simulink model "Hunter_Real_call"  (R2023a)
settings: Solver=ode3  StartTime=0.0  StopTime=inf  FixedStep=0.05  RelTol=1e-3  EnableMultiTasking=on
InitFcn:
  | rosshutdown
  | rosinit("http://localhost:11311")
model workspace (MAT data in the model file):
  SL_ROS_VariableLengthArrays_MaxSizes.CommonInfo.ArrayTruncateAction = 'EmitWarning'
  SL_ROS_VariableLengthArrays_MaxSizes.MsgTypeMap = containers.Map
  SL_ROS_VariableLengthArrays_MaxSizes.MsgTypeMap.serialization.keys = {'cob_object_detection_msgs/Detection', 'cob_object_detection_msgs/DetectionArray', 'gazebo_msgs/ModelStates', 'sensor_msgs/PointCloud2'}
  SL_ROS_VariableLengthArrays_MaxSizes.MsgTypeMap.serialization.values{1}(1).PropertyName = 'Detector'
  SL_ROS_VariableLengthArrays_MaxSizes.MsgTypeMap.serialization.values{1}(1).DataType = 'uint8'
  SL_ROS_VariableLengthArrays_MaxSizes.MsgTypeMap.serialization.values{1}(1).MaxLength = 128
  SL_ROS_VariableLengthArrays_MaxSizes.MsgTypeMap.serialization.values{1}(2).PropertyName = 'Label'
  SL_ROS_VariableLengthArrays_MaxSizes.MsgTypeMap.serialization.values{1}(2).DataType = 'uint8'
  SL_ROS_VariableLengthArrays_MaxSizes.MsgTypeMap.serialization.values{1}(2).MaxLength = 128
  SL_ROS_VariableLengthArrays_MaxSizes.MsgTypeMap.serialization.values{2}.PropertyName = 'Detections'
  SL_ROS_VariableLengthArrays_MaxSizes.MsgTypeMap.serialization.values{2}.DataType = 'cob_object_detection_msgs/Detection'
  SL_ROS_VariableLengthArrays_MaxSizes.MsgTypeMap.serialization.values{2}.MaxLength = 100
  SL_ROS_VariableLengthArrays_MaxSizes.MsgTypeMap.serialization.values{3}(1).PropertyName = 'Name'
  SL_ROS_VariableLengthArrays_MaxSizes.MsgTypeMap.serialization.values{3}(1).DataType = 'std_msgs/String'
  SL_ROS_VariableLengthArrays_MaxSizes.MsgTypeMap.serialization.values{3}(1).MaxLength = 266
  SL_ROS_VariableLengthArrays_MaxSizes.MsgTypeMap.serialization.values{3}(2).PropertyName = 'Pose'
  SL_ROS_VariableLengthArrays_MaxSizes.MsgTypeMap.serialization.values{3}(2).DataType = 'geometry_msgs/Pose'
  SL_ROS_VariableLengthArrays_MaxSizes.MsgTypeMap.serialization.values{3}(2).MaxLength = 350
  SL_ROS_VariableLengthArrays_MaxSizes.MsgTypeMap.serialization.values{3}(3).PropertyName = 'Twist'
  SL_ROS_VariableLengthArrays_MaxSizes.MsgTypeMap.serialization.values{3}(3).DataType = 'geometry_msgs/Twist'
  SL_ROS_VariableLengthArrays_MaxSizes.MsgTypeMap.serialization.values{3}(3).MaxLength = 350
  SL_ROS_VariableLengthArrays_MaxSizes.MsgTypeMap.serialization.values{4}(1).PropertyName = 'Data'
  SL_ROS_VariableLengthArrays_MaxSizes.MsgTypeMap.serialization.values{4}(1).DataType = 'uint8'
  SL_ROS_VariableLengthArrays_MaxSizes.MsgTypeMap.serialization.values{4}(1).MaxLength = 1050000
  SL_ROS_VariableLengthArrays_MaxSizes.MsgTypeMap.serialization.values{4}(2).PropertyName = 'Fields'
  SL_ROS_VariableLengthArrays_MaxSizes.MsgTypeMap.serialization.values{4}(2).DataType = 'sensor_msgs/PointField'
  SL_ROS_VariableLengthArrays_MaxSizes.MsgTypeMap.serialization.values{4}(2).MaxLength = 1000
  SL_ROS_VariableLengthArrays_MaxSizes.MsgTypeMap.serialization.uniformity = 0
  SL_ROS_VariableLengthArrays_MaxSizes.MsgTypeMap.serialization.keyType = 'char'
  SL_ROS_VariableLengthArrays_MaxSizes.MsgTypeMap.serialization.valueType = 'any'
undefined symbols (not defined in the file or in its folder): Angular, L, Ld, Linear
libraries: robotlib x10, slpidlib x2, slctrlblks x1, robotalgslib x1, mobileRoboticsLib x1, robotcorelib x1
settings Model: Creator=aiv_  LastModifiedBy=aiv
settings SolverCC: AutoInsertRateTranBlk=on
settings DataIOCC: SaveFormat=Array  ReturnWorkspaceOutputs=off
settings OptimizationCC: EnhancedBackFolding=on  PassReuseOutputArgsAs=Individual arguments  StateBitsets=on  DataBitsets=on  ZeroExternalMemoryAtStartup=off  ZeroInternalMemoryAtStartup=off  NoFixptDivByZeroProtection=on  LifeSpan=1  MaxStackSize=64  OptimizeBlockOrder=speed  DifferentSizesBufferReuse=on  EfficientTunableParamExpr=on
settings DebuggingCC: ParameterTunabilityLossMsg=error
settings HardwareCC: ProdBitPerPointer=32  ProdBitPerSizeT=32  ProdBitPerPtrDiffT=32  ProdLargestAtomicFloat=None  ProdWordSize=32  ProdHWDeviceType=Custom Processor->Custom Processor
settings ModelReferenceCC: PropagateSignalLabelsOutOfModel=off
settings SFSimCC: SimTargetLang=C++
settings RTWCC: Description=Embedded Coder  SystemTargetFile=ert.tlc  HardwareBoard=Robot Operating System (ROS)  TLCOptions=-p0 -aRateBasedStepFcn=0  TemplateMakefile=ert_default_tmf  GenerateReport=on  RTWVerbose=off  Toolchain=Catkin  IncludeHyperlinkInReport=on  LaunchReport=on  TargetLang=C++
settings CodeAppCC: ForceParamTrailComments=on  IgnoreCustomStorageClasses=off  OperatorAnnotations=on  SimulinkDataObjDesc=on  SFDataObjDesc=on  CustomSymbolStrGlobalVar=rt$N$M  CustomSymbolStrType=$N$M  CustomSymbolStrFcn=$N$M$F  CustomSymbolStrMacro=$N$M  InsertBlockDesc=on
settings ERTTargetCC: CodeReplacementLibrary=GNU C99 extensions  SuppressErrorStatus=on  CodeInterfacePackaging=C++ class  SupportVariableSizeSignals=on  RootIOFormat=Structure reference  ERTCustomFileTemplate=example_file_process.tlc

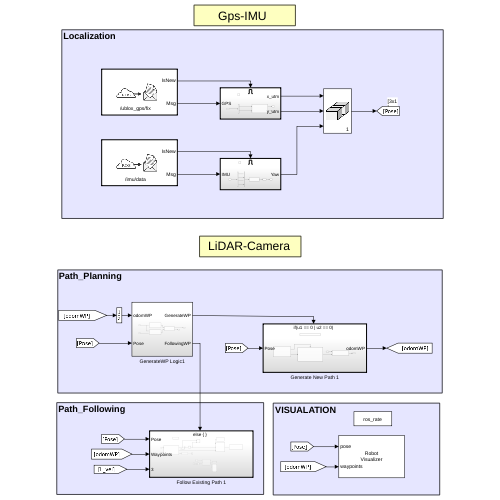
[thumbnail: Simulink's stored preview of the top-level diagram]
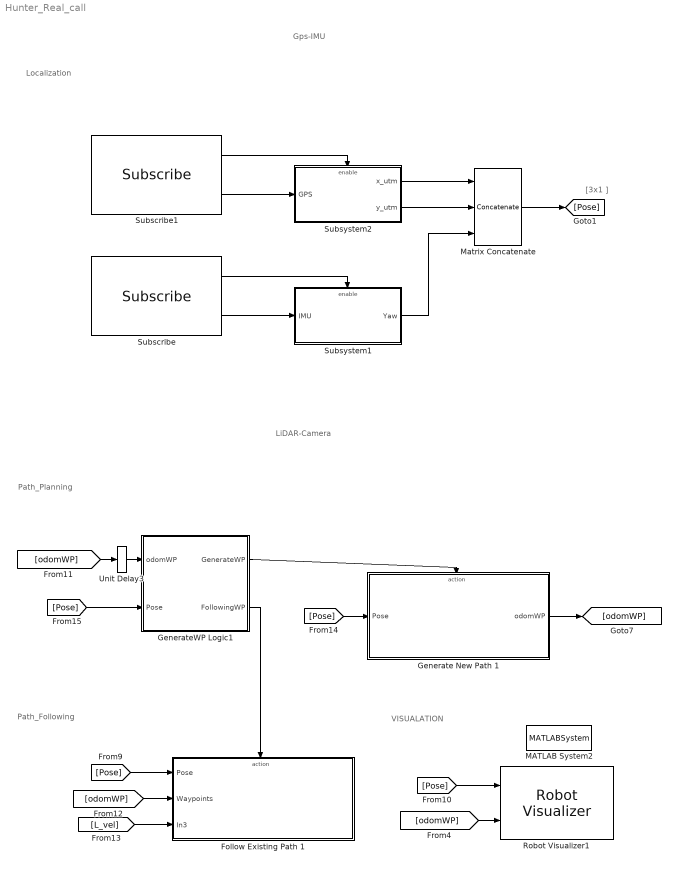
== system Hunter_Real_call ==
  note: Path_Following
  note: VISUALATION
  note: [3x1
      | ]
  note: Localization
  note: Gps-IMU
  note: LiDAR-Camera
  note: Path_Planning
  Follow Existing Path 1 : Subsystem  TreatAsAtomicUnit=on
  Generate New Path 1 : Subsystem  TreatAsAtomicUnit=on
  GenerateWP Logic1 : Subsystem
  MATLAB System2 : MATLABSystem  System=ros_rate  RATE=[20]  SimulateUsing=Code generation
      mask Type: ros_rate
      mask Display: disp('ros_rate');
  Matrix Concatenate : Concatenate  NumInputs=3  Mode=Multidimensional array
  Robot Visualizer1 : mobileRoboticsLib/Environments/Robot Visualizer  robotRadius=0  showTrajectory=on  hasWaypoints=on  hasLidar=off  sensorOffset=[ 0, 0 ]  scanAngles=[ -pi/4, 0, pi/4 ]  hasObjDetector=off  objDetectorOffset=[ 0, 0 ]  objDetectorAngle=0  objDetectorFOV=pi/4  objDetectorMaxRange=5  objectColors=[ 1, 0, 0; 0, 1, 0; 0, 0, 1 ]  objectMarkers=s
  Subscribe : robotlib/Subscribe  topicSource=Select from ROS network  topic=/imu/data  messageType=sensor_msgs/Imu  SampleTime=-1  legacyBusStruct=off  messageQueueLength=1
  Subscribe1 : robotlib/Subscribe  topicSource=Select from ROS network  topic=/ublox_gps/fix  messageType=sensor_msgs/NavSatFix  SampleTime=-1  legacyBusStruct=off  messageQueueLength=1
  Subsystem1 : Subsystem
  Subsystem2 : Subsystem
  Unit Delay3 : UnitDelay  SampleTime=-1  HasFrameUpgradeWarning=on
  wires:
  Matrix Concatenate/1 -> [Pose]
  Subsystem1/1(Yaw) -> Matrix Concatenate/3
  Subscribe/1 -> Subsystem1/Enable
  Subscribe1/2 -> Subsystem2/1(GPS)
  Subsystem2/2(y_utm) -> Matrix Concatenate/2
  Unit Delay3/1 -> GenerateWP Logic1/1(odomWP)
  [odomWP] -> Unit Delay3/1
  Subsystem2/1(x_utm) -> Matrix Concatenate/1
  [L_vel] -> Follow Existing Path 1/3(In3)
  [odomWP] -> Robot Visualizer1/2
  Subscribe1/1 -> Subsystem2/Enable
  Subscribe/2 -> Subsystem1/1(IMU)
  Generate New Path 1/1(odomWP) -> [odomWP]
  [Pose] -> GenerateWP Logic1/2(Pose)
  [Pose] -> Follow Existing Path 1/1(Pose)
  [Pose] -> Robot Visualizer1/1
  GenerateWP Logic1/1(GenerateWP) -> Generate New Path 1/Action
  [odomWP] -> Follow Existing Path 1/2(Waypoints)
  [Pose] -> Generate New Path 1/1(Pose)
  GenerateWP Logic1/2(FollowingWP) -> Follow Existing Path 1/Action

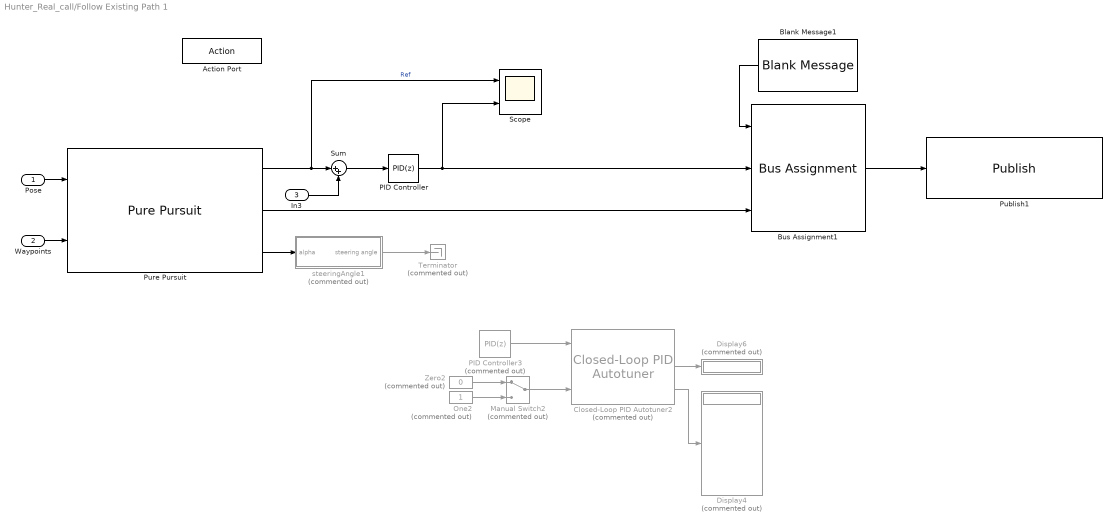
== system Hunter_Real_call/Follow Existing Path 1 ==
  Pose : Inport
  Waypoints : Inport  Port=2
  In3 : Inport  Port=3
  Action Port : ActionPort  ActionPortLabel=else
  Blank Message1 : robotlib/Blank Message  messageClass=Message  entityType=geometry_msgs/Twist  messageType=geometry_msgs/Twist  SampleTime=inf  legacyBusStruct=off
  Bus Assignment1 : BusAssignment  AssignedSignals=Linear.X,Angular.Z
  Closed-Loop PID Autotuner2 : slctrlblks/Closed-Loop PID Autotuner  Commented=on  PIDType=PID  PIDForm=Parallel  TimeDomain=discrete-time  DiscreteTs=0.05  TuningTs=0.2  UseTuningTs=off  IntegratorFormula=Forward Euler  FilterFormula=Forward Euler  ContinuousTs=0.02  Bandwidth=1  UseExternalWC=off  TargetPM=60  UseExternalPM=off  UseExternalAchievedPM=off  ExperimentMode=Superposition  PlantType=Stable  PlantSign=Positive  AmpSine=0.01  UseExternalAmpSine=off  UseExternalFRD=off  UseExternalU0=off  UseCompanion=off  NotDeployTuningModule=off  UsePLCCoder=off  OutputMode=control action + perturbation  BlockDataType=double  UseConnectedPID=on  blockpath=[]  tunedP=0  tunedI=0  tunedD=0  tunedN=100  tunedPM=0  EstimationWindowSize=3  UseExternalTuningParams=off  SingleMultiRateVariant=SingleSamplingRate  NumEstimationPeriods=4  NumSettlingPeriods=2  ExperimentModeVariant=VariantSuperimposed  OutputChoice=VariantCandD
  Display4 : Display  Commented=on
  Display6 : Display  Commented=on
  Manual Switch2 : ManualSwitch  Commented=on
  One2 : Constant  Commented=on  OutDataTypeStr=Inherit: Inherit via back propagation
  PID Controller : slpidlib/PID Controller  Controller=PID  Form=Parallel  TimeDomain=Discrete-time  UseExternalTs=off  SampleTime=-1  IntegratorMethod=Forward Euler  FilterMethod=Forward Euler  ControllerParametersSource=internal  P=0.3475  I=0.1757  UseKiTs=off  D=0  N=100  UseFilter=on  TunerSelectOption=Transfer Function Based (PID Tuner App)  InitialConditionSource=internal  InitialConditionForIntegrator=0  InitialConditionForFilter=0  DifferentiatorICPrevScaledInput=0  ExternalReset=none  TrackingMode=off  Kt=1  LimitOutput=off  SatLimitsSource=internal  UpperSaturationLimit=inf  LowerSaturationLimit=-inf  LinearizeAsGain=on  AntiWindupMode=none  Kb=1  LimitIntegrator=off  UpperIntegratorSaturationLimit=inf  LowerIntegratorSaturationLimit=-inf  POutMin=[]  POutMax=[]  IOutMin=[]  IOutMax=[]  DOutMin=[]  DOutMax=[]  NOutMin=[]  NOutMax=[]  SumOutMin=[]  SumOutMax=[]  SaturationOutMin=[]  SaturationOutMax=[]  PParamMin=[]  PParamMax=[]  IParamMin=[]  IParamMax=[]  DParamMin=[]  DParamMax=[]  NParamMin=[]  NParamMax=[]  KbParamMin=[]  KbParamMax=[]  KtParamMin=[]  KtParamMax=[]  KbOutMin=[]  KbOutMax=[]  KtOutMin=[]  KtOutMax=[]  IntegratorOutMin=[]  IntegratorOutMax=[]  FilterOutMin=[]  FilterOutMax=[]  SumI1OutMin=[]  SumI1OutMax=[]  SumI2OutMin=[]  SumI2OutMax=[]  SumI3OutMin=[]  SumI3OutMax=[]  SumI4OutMin=[]  SumI4OutMax=[]  SumDOutMin=[]  SumDOutMax=[]  DifferentiatorOutMin=[]  DifferentiatorOutMax=[]  FilterDiffOutCoefMin=[]  FilterDiffOutCoefMax=[]  ReciprocalOutMin=[]  ReciprocalOutMax=[]  SumDenOutMin=[]  SumDenOutMax=[]  SumNumOutMin=[]  SumNumOutMax=[]  DivideOutMin=[]  DivideOutMax=[]  UdiffTsProdOutMin=[]  UdiffTsProdOutMax=[]  NTsProdOutMin=[]  NTsProdOutMax=[]  UintegralTsProdOutMin=[]  UintegralTsProdOutMax=[]  UngainTsProdOutMin=[]  UngainTsProdOutMax=[]  ClampingZeroOutDataTypeStr=Inherit: Inherit via back propagation  ClampingZeroOutMin=[]  ClampingZeroOutMax=[]  FilterDenConstantOutDataTypeStr=Inherit: Inherit via back propagation  FilterDenConstantOutMin=[]  FilterDenConstantOutMax=[]  PCopyOutDataTypeStr=Inherit: Inherit via back propagation  PCopyOutMin=[]  PCopyOutMax=[]  NCopyOutDataTypeStr=Inherit: Inherit via back propagation  NCopyOutMin=[]  NCopyOutMax=[]  IntegratorContinuousStateAttributes=''  IntegratorStateMustResolveToSignalObject=off  IntegratorRTWStateStorageClass=Auto  FilterContinuousStateAttributes=''  FilterStateMustResolveToSignalObject=off  FilterRTWStateStorageClass=Auto  ParallelPVariant=InternalParameters  IdealPVariant=Disabled  IVariant=InternalParameters  DVariant=InternalParameters  IntegratorVariant=Discrete  SatVariant=Disabled  AWVariant=Passthrough  PCopyVariant=Disabled  TRVariant=Disabled  FdbkBlocksVariant=Forward  IdealPFdbkVariant=Disabled  SatFdbkVariant=Disabled  DerivativeFilterVariant=ForwardEulerFilter  NVariant=InternalParameters  NCopyVariant=Disabled  FilterICVariant=InternalICsFilter  IntegratorICVariant=InternalICs  ExternalResetVariant=Disabled  TRSumVariant=Passthrough  SumFdbkVariant=Disabled  SumVariant=Sum_PID  TsampFilterVariant=InternalTs  TsampNgainVariant=Passthrough  TsampIntegralVariant=Disabled_SignalSpec  ExternalSaturationOutDataTypeStr=Inherit: Same as second input
  PID Controller3 : slpidlib/PID Controller  Commented=on  Controller=PID  Form=Parallel  TimeDomain=Discrete-time  UseExternalTs=off  SampleTime=-1  IntegratorMethod=Forward Euler  FilterMethod=Forward Euler  ControllerParametersSource=internal  P=1  I=1  UseKiTs=off  D=0  N=100  UseFilter=on  TunerSelectOption=Transfer Function Based (PID Tuner App)  InitialConditionSource=internal  InitialConditionForIntegrator=0  InitialConditionForFilter=0  DifferentiatorICPrevScaledInput=0  ExternalReset=none  TrackingMode=off  Kt=1  LimitOutput=off  SatLimitsSource=internal  UpperSaturationLimit=inf  LowerSaturationLimit=-inf  LinearizeAsGain=on  AntiWindupMode=none  Kb=1  LimitIntegrator=off  UpperIntegratorSaturationLimit=inf  LowerIntegratorSaturationLimit=-inf  POutMin=[]  POutMax=[]  IOutMin=[]  IOutMax=[]  DOutMin=[]  DOutMax=[]  NOutMin=[]  NOutMax=[]  SumOutMin=[]  SumOutMax=[]  SaturationOutMin=[]  SaturationOutMax=[]  PParamMin=[]  PParamMax=[]  IParamMin=[]  IParamMax=[]  DParamMin=[]  DParamMax=[]  NParamMin=[]  NParamMax=[]  KbParamMin=[]  KbParamMax=[]  KtParamMin=[]  KtParamMax=[]  KbOutMin=[]  KbOutMax=[]  KtOutMin=[]  KtOutMax=[]  IntegratorOutMin=[]  IntegratorOutMax=[]  FilterOutMin=[]  FilterOutMax=[]  SumI1OutMin=[]  SumI1OutMax=[]  SumI2OutMin=[]  SumI2OutMax=[]  SumI3OutMin=[]  SumI3OutMax=[]  SumI4OutMin=[]  SumI4OutMax=[]  SumDOutMin=[]  SumDOutMax=[]  DifferentiatorOutMin=[]  DifferentiatorOutMax=[]  FilterDiffOutCoefMin=[]  FilterDiffOutCoefMax=[]  ReciprocalOutMin=[]  ReciprocalOutMax=[]  SumDenOutMin=[]  SumDenOutMax=[]  SumNumOutMin=[]  SumNumOutMax=[]  DivideOutMin=[]  DivideOutMax=[]  UdiffTsProdOutMin=[]  UdiffTsProdOutMax=[]  NTsProdOutMin=[]  NTsProdOutMax=[]  UintegralTsProdOutMin=[]  UintegralTsProdOutMax=[]  UngainTsProdOutMin=[]  UngainTsProdOutMax=[]  ClampingZeroOutDataTypeStr=Inherit: Inherit via back propagation  ClampingZeroOutMin=[]  ClampingZeroOutMax=[]  FilterDenConstantOutDataTypeStr=Inherit: Inherit via back propagation  FilterDenConstantOutMin=[]  FilterDenConstantOutMax=[]  PCopyOutDataTypeStr=Inherit: Inherit via back propagation  PCopyOutMin=[]  PCopyOutMax=[]  NCopyOutDataTypeStr=Inherit: Inherit via back propagation  NCopyOutMin=[]  NCopyOutMax=[]  IntegratorContinuousStateAttributes=''  IntegratorStateMustResolveToSignalObject=off  IntegratorRTWStateStorageClass=Auto  FilterContinuousStateAttributes=''  FilterStateMustResolveToSignalObject=off  FilterRTWStateStorageClass=Auto  ParallelPVariant=InternalParameters  IdealPVariant=Disabled  IVariant=InternalParameters  DVariant=InternalParameters  IntegratorVariant=Discrete  SatVariant=Disabled  AWVariant=Passthrough  PCopyVariant=Disabled  TRVariant=Disabled  FdbkBlocksVariant=Forward  IdealPFdbkVariant=Disabled  SatFdbkVariant=Disabled  DerivativeFilterVariant=ForwardEulerFilter  NVariant=InternalParameters  NCopyVariant=Disabled  FilterICVariant=InternalICsFilter  IntegratorICVariant=InternalICs  ExternalResetVariant=Disabled  TRSumVariant=Passthrough  SumFdbkVariant=Disabled  SumVariant=Sum_PID  TsampFilterVariant=InternalTs  TsampNgainVariant=Passthrough  TsampIntegralVariant=Disabled_SignalSpec  ExternalSaturationOutDataTypeStr=Inherit: Same as second input
  Publish1 : robotlib/Publish  topicSource=Select from ROS network  topic=/ackermann_steering_controller/cmd_vel  messageType=geometry_msgs/Twist  legacyBusStruct=off  messageQueueLength=1
  Pure Pursuit : robotalgslib/Pure Pursuit  DesiredLinearVelocity=1.5  MaxAngularVelocity=2  LookaheadDistance=1.3  TargetDirPort=on  SimulateUsing=Code generation
      settings: LibrarySourceBlock=navlib/Control Algorithms/Pure Pursuit
  Scope : Scope  NumInputPorts=2
  Sum : Sum  Inputs=|++
  Terminator : Terminator  Commented=on
  Zero2 : Constant  Commented=on  Value=0  OutDataTypeStr=Inherit: Inherit via back propagation
  steeringAngle1 : Subsystem  Commented=on
  wires:
  Pose/1 -> Pure Pursuit/1
  Waypoints/1 -> Pure Pursuit/2
  Bus Assignment1/1 -> Publish1/1
  Blank Message1/1 -> Bus Assignment1/1
  Pure Pursuit/3 -> steeringAngle1/1(alpha)
  Pure Pursuit/2 -> Bus Assignment1/3
  PID Controller/1 -> Scope/2, Bus Assignment1/2
  Sum/1 -> PID Controller/1
  Pure Pursuit/1 -> Scope/1, Sum/1  "Ref"
  In3/1 -> Sum/2
  PID Controller3/1 -> Closed-Loop PID Autotuner2/1
  Manual Switch2/1 -> Closed-Loop PID Autotuner2/3
  Closed-Loop PID Autotuner2/3 -> Display4/1
  Zero2/1 -> Manual Switch2/1
  Closed-Loop PID Autotuner2/2 -> Display6/1
  One2/1 -> Manual Switch2/2
  steeringAngle1/1(steering angle) -> Terminator/1

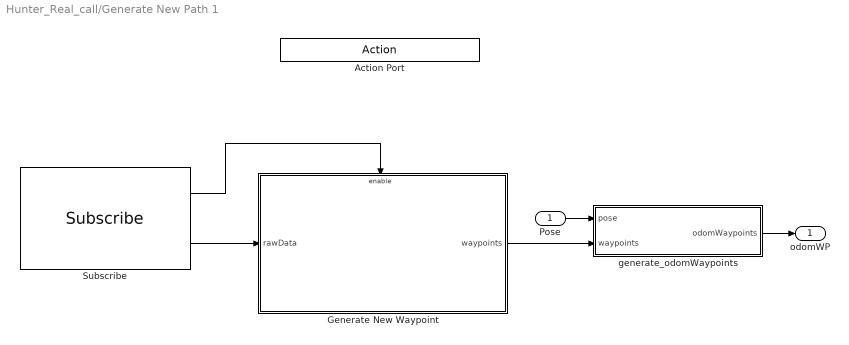
== system Hunter_Real_call/Generate New Path 1 ==
  Pose : Inport
  Action Port : ActionPort  PropagateVarSize=During execution  ActionPortLabel=if(u1 == 0 | u2 == 0)
  Generate New Waypoint : Subsystem
  Subscribe : robotlib/Subscribe  topicSource=Select from ROS network  topic=/lidar  messageType=sensor_msgs/PointCloud2  SampleTime=-1  legacyBusStruct=off  messageQueueLength=1
  generate_odomWaypoints : MATLAB Function  TreatAsAtomicUnit=on
  odomWP : Outport
  wires:
  Subscribe/2 -> Generate New Waypoint/1(rawData)
  generate_odomWaypoints/1(odomWaypoints) -> odomWP/1
  Subscribe/1 -> Generate New Waypoint/Enable
  Pose/1 -> generate_odomWaypoints/1(pose)
  Generate New Waypoint/1(waypoints) -> generate_odomWaypoints/2(waypoints)

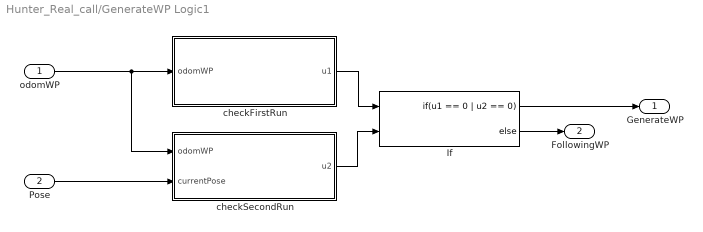
== system Hunter_Real_call/GenerateWP Logic1 ==
  odomWP : Inport
  Pose : Inport  Port=2
  If : If  NumInputs=2  IfExpression=u1 == 0 | u2 == 0
  checkFirstRun : MATLAB Function  TreatAsAtomicUnit=on
  checkSecondRun : MATLAB Function  TreatAsAtomicUnit=on
  GenerateWP : Outport
  FollowingWP : Outport  Port=2
  wires:
  checkSecondRun/1(u2) -> If/2
  odomWP/1 -> checkSecondRun/1(odomWP), checkFirstRun/1(odomWP)
  If/2 -> FollowingWP/1
  checkFirstRun/1(u1) -> If/1
  Pose/1 -> checkSecondRun/2(currentPose)
  If/1 -> GenerateWP/1

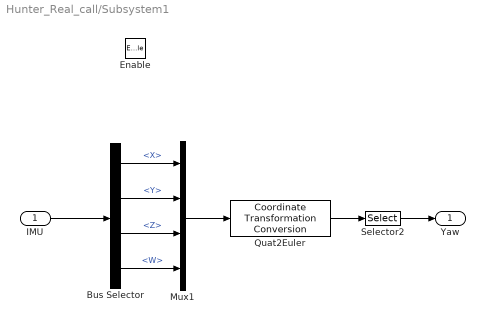
== system Hunter_Real_call/Subsystem1 ==
  IMU : Inport
  Enable : EnablePort
  Bus Selector : BusSelector  OutputSignals=Orientation.X,Orientation.Y,Orientation.Z,Orientation.W
  Mux1 : Mux
  Quat2Euler : robotcorelib/Coordinate Transformation Conversion  InputRepresentation=Quaternion  InputEulerSequence=ZYX  ShowTrVecInputPort=on  OutputRepresentation=Euler Angles  OutputEulerSequence=ZYX  ShowTrVecOutputPort=on  SimulateUsing=Interpreted execution
  Selector2 : Selector  InputPortWidth=3  IndexOptions=Index vector (dialog)  Indices=3  OutputSizes=1
  Yaw : Outport
  wires:
  IMU/1 -> Bus Selector/1
  Mux1/1 -> Quat2Euler/1
  Bus Selector/1 -> Mux1/1  "<X>"
  Bus Selector/2 -> Mux1/2  "<Y>"
  Bus Selector/3 -> Mux1/3  "<Z>"
  Bus Selector/4 -> Mux1/4  "<W>"
  Quat2Euler/1 -> Selector2/1
  Selector2/1 -> Yaw/1

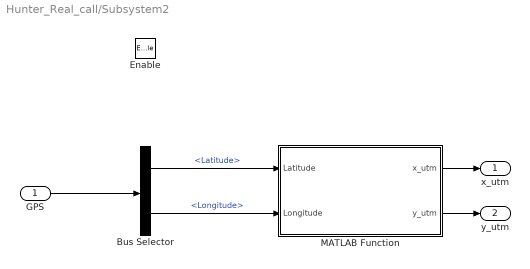
== system Hunter_Real_call/Subsystem2 ==
  GPS : Inport
  Enable : EnablePort
  Bus Selector : BusSelector  OutputSignals=Latitude,Longitude
  MATLAB Function : MATLAB Function  TreatAsAtomicUnit=on
  x_utm : Outport
  y_utm : Outport  Port=2
  wires:
  GPS/1 -> Bus Selector/1
  Bus Selector/1 -> MATLAB Function/1(Latitude)  "<Latitude>"
  Bus Selector/2 -> MATLAB Function/2(Longitude)  "<Longitude>"
  MATLAB Function/1(x_utm) -> x_utm/1
  MATLAB Function/2(y_utm) -> y_utm/1

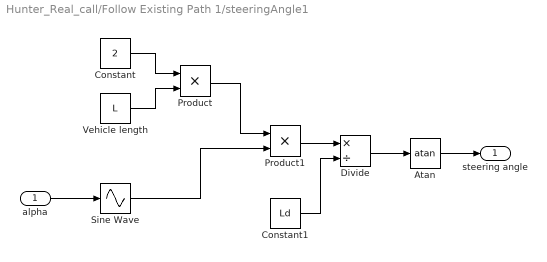
== system Hunter_Real_call/Follow Existing Path 1/steeringAngle1 ==
  alpha : Inport
  Atan : Trigonometry  Operator=atan
  Constant : Constant  Value=2
  Constant1 : Constant  Value=Ld
  Divide : Product  Inputs=*/
  Product : Product
  Product1 : Product
  Sine Wave : Sin  TimeSource=Use external signal  SampleTime=0
  Vehicle length : Constant  Value=L
  steering angle : Outport
  wires:
  Constant/1 -> Product/1
  Vehicle length/1 -> Product/2
  alpha/1 -> Sine Wave/1
  Product/1 -> Product1/1
  Sine Wave/1 -> Product1/2
  Product1/1 -> Divide/1
  Constant1/1 -> Divide/2
  Divide/1 -> Atan/1
  Atan/1 -> steering angle/1

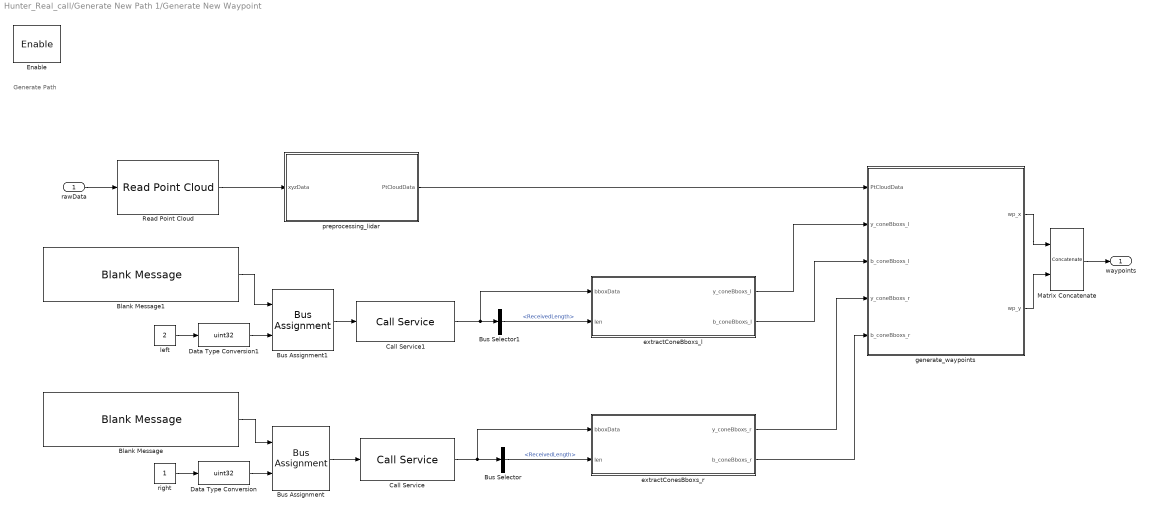
== system Hunter_Real_call/Generate New Path 1/Generate New Waypoint ==
  note: Generate Path
  rawData : Inport
  Enable : EnablePort  PropagateVarSize=During execution
  Blank Message : robotlib/Blank Message  messageClass=Service Request  entityType=cob_object_detection_msgs/DetectObjects  messageType=cob_object_detection_msgs/DetectObjectsRequest  SampleTime=inf  legacyBusStruct=off
  Blank Message1 : robotlib/Blank Message  messageClass=Service Request  entityType=cob_object_detection_msgs/DetectObjects  messageType=cob_object_detection_msgs/DetectObjectsRequest  SampleTime=inf  legacyBusStruct=off
  Bus Assignment : BusAssignment  AssignedSignals=Roi.Height
  Bus Assignment1 : BusAssignment  AssignedSignals=Roi.Height
  Bus Selector : BusSelector  OutputSignals=ObjectList.Detections_SL_Info.ReceivedLength
  Bus Selector1 : BusSelector  OutputSignals=ObjectList.Detections_SL_Info.ReceivedLength
  Call Service : robotlib/Call Service  topicSource=Specify your own  service=/Activate_yolo  serviceType=cob_object_detection_msgs/DetectObjects  connectionTimeout=5  keepPersistent=off  ShowErrorCodeOutput=off  legacyBusStruct=off
  Call Service1 : robotlib/Call Service  topicSource=Specify your own  service=/Activate_yolo  serviceType=cob_object_detection_msgs/DetectObjects  connectionTimeout=5  keepPersistent=off  ShowErrorCodeOutput=off  legacyBusStruct=off
  Data Type Conversion : DataTypeConversion  OutDataTypeStr=uint32  SaturateOnIntegerOverflow=off  RndMeth=Floor
  Data Type Conversion1 : DataTypeConversion  OutDataTypeStr=uint32  SaturateOnIntegerOverflow=off  RndMeth=Floor
  Matrix Concatenate : Concatenate  Mode=Multidimensional array  ConcatenateDimension=2
  Read Point Cloud : robotlib/Read Point Cloud  MaximumPointCloudSize=[1, 32768]  PreserveStructure=on  ShowRGBOutput=off  ShowIntensityOutput=off  ShowErrorCodeOutput=off  VariableSizeOutputs=off
  extractConeBboxs_l : MATLAB Function  TreatAsAtomicUnit=on
  extractConesBboxs_r : MATLAB Function  TreatAsAtomicUnit=on
  generate_waypoints : MATLAB Function  TreatAsAtomicUnit=on
  left : Constant  Value=2
  preprocessing_lidar : MATLAB Function  TreatAsAtomicUnit=on
  right : Constant
  waypoints : Outport
  wires:
  rawData/1 -> Read Point Cloud/1
  Read Point Cloud/1 -> preprocessing_lidar/1(xyzData)
  Call Service/1 -> Bus Selector/1, extractConesBboxs_r/1(bboxData)
  right/1 -> Data Type Conversion/1
  Bus Assignment1/1 -> Call Service1/1
  Data Type Conversion/1 -> Bus Assignment/2
  Blank Message1/1 -> Bus Assignment1/1
  left/1 -> Data Type Conversion1/1
  Call Service1/1 -> extractConeBboxs_l/1(bboxData), Bus Selector1/1
  Bus Selector1/1 -> extractConeBboxs_l/2(len)  "<ReceivedLength>"
  Bus Selector/1 -> extractConesBboxs_r/2(len)  "<ReceivedLength>"
  Bus Assignment/1 -> Call Service/1
  Data Type Conversion1/1 -> Bus Assignment1/2
  Blank Message/1 -> Bus Assignment/1
  extractConeBboxs_l/1(y_coneBboxs_l) -> generate_waypoints/2(y_coneBboxs_l)
  extractConeBboxs_l/2(b_coneBboxs_l) -> generate_waypoints/3(b_coneBboxs_l)
  preprocessing_lidar/1(PtCloudData) -> generate_waypoints/1(PtCloudData)
  extractConesBboxs_r/1(y_coneBboxs_r) -> generate_waypoints/4(y_coneBboxs_r)
  extractConesBboxs_r/2(b_coneBboxs_r) -> generate_waypoints/5(b_coneBboxs_r)
  generate_waypoints/1(wp_x) -> Matrix Concatenate/1
  generate_waypoints/2(wp_y) -> Matrix Concatenate/2
  Matrix Concatenate/1 -> waypoints/1

== matlab function Hunter_Real_call/Generate New Path 1/Generate New Waypoint/extractConesBboxs_r ==
  data: y_coneBboxs_r output size=[50 4]; bboxData input; len input; b_coneBboxs_r output size=[50 4]
function [y_coneBboxs_r,b_coneBboxs_r] = extractConesBboxs_r(bboxData, len)

    temp_y_coneBboxs = zeros(len,4);
    temp_b_coneBboxs = zeros(len,4);

    y_count = 0;
    b_count = 0;

    % disp(len)
    for i = 1:len
        x = bboxData.ObjectList.Detections(i).Mask.Roi.X;
        y = bboxData.ObjectList.Detections(i).Mask.Roi.Y;
        w = bboxData.ObjectList.Detections(i).Mask.Roi.Width;
        h = bboxData.ObjectList.Detections(i).Mask.Roi.Height;

        label = char(bboxData.ObjectList.Detections(i).Label)';
        label = label(:,1:6);
        
        if strcmp(label,'y_cone')
            y_count = y_count + 1;
            temp_y_coneBboxs(y_count,:) = [x y w h];
        elseif strcmp(label,'b_cone')
            b_count = b_count + 1;
            temp_b_coneBboxs(b_count,:) = [x y w h];
        else
            disp("No");
        end
    end
   
    y_coneBboxs_r = temp_y_coneBboxs(1:y_count, :);
    b_coneBboxs_r = temp_b_coneBboxs(1:b_count, :);
   
end

== matlab function Hunter_Real_call/Generate New Path 1/Generate New Waypoint/extractConeBboxs_l ==
  data: y_coneBboxs_l output size=[50 4]; bboxData input; len input; b_coneBboxs_l output size=[50 4]
function [y_coneBboxs_l, b_coneBboxs_l] = extractConesBboxs_l(bboxData, len)

    temp_y_coneBboxs = zeros(len,4);
    temp_b_coneBboxs = zeros(len,4);

    y_count = 0;
    b_count = 0;

    % disp(len)
    for i = 1:len
        x = bboxData.ObjectList.Detections(i).Mask.Roi.X;
        y = bboxData.ObjectList.Detections(i).Mask.Roi.Y;
        w = bboxData.ObjectList.Detections(i).Mask.Roi.Width;
        h = bboxData.ObjectList.Detections(i).Mask.Roi.Height;

        label = char(bboxData.ObjectList.Detections(i).Label)';
        label = label(:,1:6);
        
        if strcmp(label,'y_cone')
            y_count = y_count + 1;
            temp_y_coneBboxs(y_count,:) = [x y w h];
        elseif strcmp(label,'b_cone')
            b_count = b_count + 1;
            temp_b_coneBboxs(b_count,:) = [x y w h];
        else
            disp("No");
        end
    end
   
    y_coneBboxs_l = temp_y_coneBboxs(1:y_count, :);
    b_coneBboxs_l = temp_b_coneBboxs(1:b_count, :);
   
end

== matlab function Hunter_Real_call/Subsystem2/MATLAB Function ==
  data: Latitude input; x_utm output; Longitude input; y_utm output
function [x_utm, y_utm] =convertUTM(Latitude, Longitude)

    [x_utm, y_utm] = projfwd(projcrs(32652),Latitude,Longitude);

end

== matlab function Hunter_Real_call/Generate New Path 1/Generate New Waypoint/generate_waypoints ==
  data: PtCloudData input single size=[3000 3]; y_coneBboxs_l input; b_coneBboxs_l input; y_coneBboxs_r input; b_coneBboxs_r input; wp_x output size=[50,1]; wp_y output size=[50,1]
function [wp_x, wp_y] = generate_waypoints(PtCloudData, y_coneBboxs_l, b_coneBboxs_l,y_coneBboxs_r, b_coneBboxs_r)      
    %#codegen
    coder.extrinsic("generateWaypoints");
    wp_x = double(zeros(50,1));
    wp_y = double(zeros(50,1));

    [wp_x, wp_y] = generateWaypoints(PtCloudData,...
                                     y_coneBboxs_l, b_coneBboxs_l,...
                                     y_coneBboxs_r, b_coneBboxs_r);
end

== matlab function Hunter_Real_call/Generate New Path 1/Generate New Waypoint/preprocessing_lidar ==
  data: xyzData input single; PtCloudData output size=[3000 3]
function PtCloudData = preprocessing_lidar(xyzData)
    % waypoint_x, waypoint_y
    %% preprocessing raw lidar data
    params = lidarParameters('OS1Gen1-64',512);
    roi = [0, 7, -7, 7, -1, 2];

    ptCloud = pointCloud(xyzData);
    ptCloudOrg = pcorganize(ptCloud,params);
    
    groundPtIdx = segmentGroundFromLidarData(ptCloudOrg);
    nonGroundPtCloud = select(ptCloudOrg,~groundPtIdx,'OutputSize','full');
    
    indices = findPointsInROI(nonGroundPtCloud,roi);
    roiPtCloud = select(nonGroundPtCloud,indices);

    roiPtCloud = pcdenoise(roiPtCloud,"PreserveStructure",true);
    PtCloudData = roiPtCloud.Location;
    
end

== matlab function Hunter_Real_call/Generate New Path 1/generate_odomWaypoints ==
  data: pose input; waypoints input; odomWaypoints output double size=[50,2]
function odomWaypoints = fcn(pose, waypoints)
    % pose [3x1] 
    % waypoints [1x2]
    
    % Initialize transformed waypoints
    odomWaypoints = zeros(size(waypoints));
    % odomWaypoints = zeros(3,2);
    
    % Extract the vehicle's yaw angle
    theta = pose(3);

    % Create the 2D rotation matrix
    R = [cos(theta), -sin(theta);
         sin(theta), cos(theta)];

    % Transform each waypoint
    for i = 1:size(waypoints,1)
        % Rotate the waypoint considering the vehicle's yaw
        rotatedPoint = R * waypoints(i,:)';

        % Translate considering the vehicle's position in the odom frame
        odomWaypoints(i,:) = rotatedPoint' + pose(1:2)';
    end
    
    
end

== matlab function Hunter_Real_call/GenerateWP Logic1/checkFirstRun ==
  data: odomWP input; u1 output
function u1 = checkWP(odomWP)
    
        
    if isempty(find(odomWP)) 
        u1 = 0;  % generate new waypoint
    else
        u1 = 1;  % follow existing waypoint
    end

end

== matlab function Hunter_Real_call/GenerateWP Logic1/checkSecondRun ==
  data: odomWP input; u2 output; currentPose input
function u2 = checkDist(odomWP, currentPose)

   if norm(odomWP(end,:) - [currentPose(1) currentPose(2)]) < 2
       u2 = 0;  % generate new waypoints
   else
       u2 = 1;  % follow existing waypoints
   end
